simulink model "model_dryden"  (R2023a)
settings: Solver=FixedStepAuto  StartTime=0.0  StopTime=t(end)  FixedStep=dt  RelTol=1e-3
values from neighbouring files (symbols this model uses):
  dt = t(2) - t(1)    [test.m]    (also in test_dryden.m = 0.001)
  seed = [23341 23342 23343 23344]    [test_dryden.m]
undefined symbols (not defined in the file or in its folder): F, Light, MIL
libraries: aerolibwind2 x1, aerolibcommonsys x1
settings Model: PauseTimes=0.001  Creator=hacs  LastModifiedBy=hacs

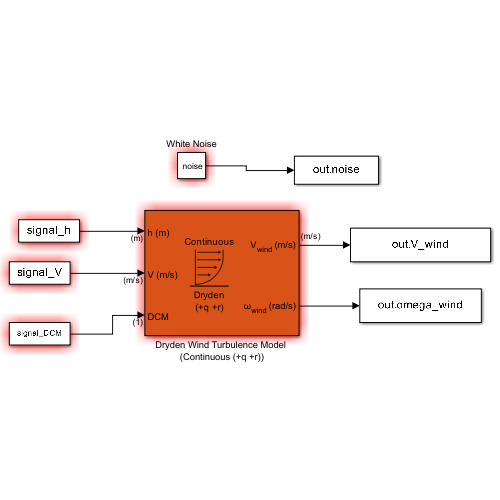
[thumbnail: Simulink's stored preview of the top-level diagram]
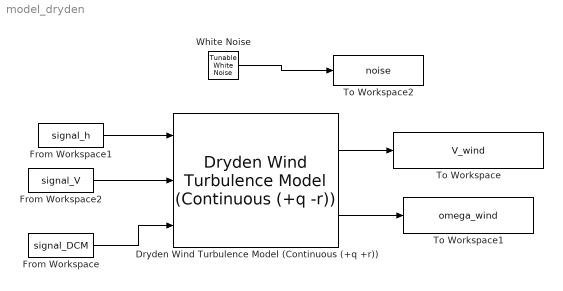
== system model_dryden ==
  Dryden Wind Turbulence Model (Continuous (+q +r)) : aerolibwind2/Dryden Wind Turbulence Model  (Continuous (+q -r))  units=Metric (MKS)  spec=MIL-F-8785C  model=Continuous Dryden (+q +r)  W20=V_wind_at6m  Wdeg=angle_wind_at6m  TurbProb=10^-2 - Light  L_high=scale_length_med  Wingspan=wingspan  ts=dt  Seed=seed  T_on=on
  From Workspace : FromWorkspace  VariableName=signal_DCM
  From Workspace1 : FromWorkspace  VariableName=signal_h
  From Workspace2 : FromWorkspace  VariableName=signal_V
  To Workspace : ToWorkspace  VariableName=V_wind  SaveFormat=Timeseries  SampleTime=-1
  To Workspace1 : ToWorkspace  VariableName=omega_wind  SaveFormat=Timeseries  SampleTime=-1
  To Workspace2 : ToWorkspace  VariableName=noise  SaveFormat=Timeseries  SampleTime=-1
  White Noise : aerolibcommonsys/Tunable White Noise  pwr=[1 1 1 1]*pi  Ts=dt  seed=seed
  wires:
  From Workspace1/1 -> Dryden Wind Turbulence Model (Continuous (+q +r))/1
  From Workspace2/1 -> Dryden Wind Turbulence Model (Continuous (+q +r))/2
  Dryden Wind Turbulence Model (Continuous (+q +r))/1 -> To Workspace/1
  From Workspace/1 -> Dryden Wind Turbulence Model (Continuous (+q +r))/3
  Dryden Wind Turbulence Model (Continuous (+q +r))/2 -> To Workspace1/1
  White Noise/1 -> To Workspace2/1
